simulink model "butter_test"  (R2020b)
settings: Solver=FixedStepAuto  StartTime=0.0  StopTime=0.00001  RelTol=1e-3
libraries: dsparch4 x1
settings Model: Creator=pablo  LastModifiedBy=pablo

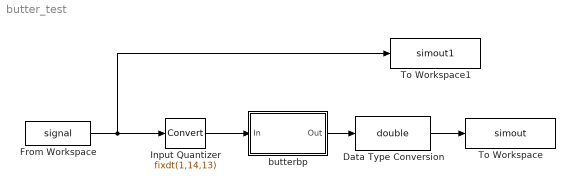
== system butter_test ==
  Data Type Conversion : DataTypeConversion  OutDataTypeStr=double
  From Workspace : FromWorkspace  VariableName=signal
  Input Quantizer : DataTypeConversion  OutDataTypeStr=fixdt(1,14,13)  RndMeth=Round  SaturateOnIntegerOverflow=on
  To Workspace : ToWorkspace  VariableName=simout  SampleTime=-1
  To Workspace1 : ToWorkspace  VariableName=simout1  SampleTime=-1
  butterbp : Subsystem  Tag=BlockMethodSubSystem
  wires:
  From Workspace/1 -> Input Quantizer/1, To Workspace1/1
  Data Type Conversion/1 -> To Workspace/1
  butterbp/1(Out) -> Data Type Conversion/1
  Input Quantizer/1 -> butterbp/1(In)

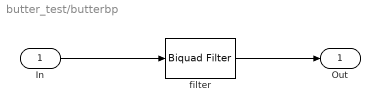
== system butter_test/butterbp ==
  In : Inport
  filter : dsparch4/Biquad Filter  FilterSource=Dialog parameters  CoeffSource=Specify via dialog  FilterObject=BQF  IIRFiltStruct=Direct form II  BiQuadCoeffs=[1 0 -1 1 -1.60137133706940249 0.992507630825395504;1 0 -1 1 -1.62252630353837413 0.992689665899144646;1 0 -1 1 -1.59926077751646867 0.982133309763404405;1 0 -1 1 -1.60806350104833395 0.982313500850860999]  ScaleValues=[0.00967072626983317592;0.00967072626983317592;0.0096206923413178231;0.0096206923413178231;1]  IC=0  ICnum=0  ICden=0  a0Flag=Warning  optimizeScaleValues=on  ScaleValueMode=Specify via input port (g)  InputProcessing=Columns as channels (frame based)  roundingMode=Convergent  overflowMode=off  stageInputMode=Binary point scaling  stageInputWordLength=16  stageInputFracLength=16  stageOutputMode=Binary point scaling  stageOutputWordLength=16  stageOutputFracLength=11  firstCoeffMode=Binary point scaling  firstCoeffWordLength=16  firstCoeffFracLength=14  scaleValueFracLength=21  prodOutputMode=Binary point scaling  prodOutputWordLength=32  prodOutputFracLength=29  denProdOutputFracLength=29  accumMode=Binary point scaling  accumWordLength=40  accumFracLength=29  denAccumFracLength=29  memoryMode=Binary point scaling  memoryWordLength=16  memoryFracLength=15  secondMemoryFracLength=15  outputMode=Binary point scaling  outputWordLength=18  outputFracLength=13
  Out : Outport
  wires:
  In/1 -> filter/1
  filter/1 -> Out/1
